simulink model "BMS_System_Arch"  (R2024a)
settings: Solver=VariableStepAuto  StartTime=0.0  StopTime=10.0  RelTol=1e-3
settings Model: DataDictionary=BMS_System_Arch_dict.sldd  Creator=ghourabi  LastModifiedBy=hirah

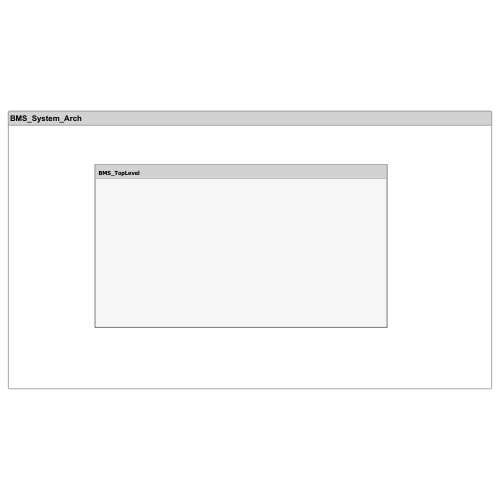
[thumbnail: Simulink's stored preview of the top-level diagram]
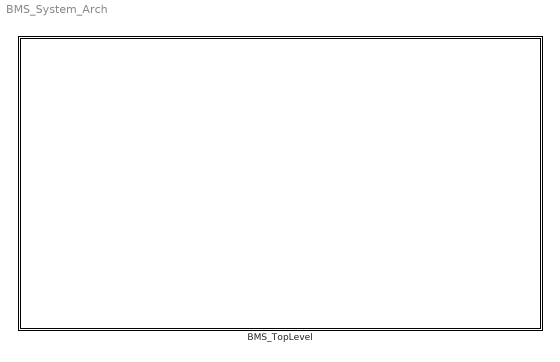
== system BMS_System_Arch ==
  "BMS_TopLevel " : Subsystem
      settings: PortSchema="{\"entries\":[{\"content\":{\"headerSize\":26,\"margin\":15,\"minimumSpacing\":25,\"sides\":[{\"content\":{},\"type\":\"ConnectorPlacement.EquallySpacedRectSide\",\"uuid\":\"3cb385af-e70b-4c78-b84b-8b5b4c1bf807\"},{\"content\":{\"side\":\"RIGHT\"},\"type\":\"ConnectorPlacement.EquallySpacedRectSide\",\"uuid\":\"e6b0f49b-5901-429a-bf04-96c47fe1d754\"},{\"content\":{\"side\":\"TOP\"},\"type\":\"ConnectorPlacement.EquallySpacedRectSide\",\"uuid\":\"0aec474f-0a8e-4cc4-a707-3f6b1e91156f\"}]},\"type\":\"ConnectorPlacement.EquallySpacedConnector\",\"uuid\":\"d23b7e1f-ccd0-4a91-b27d-bb01c8043b47\"}],\"packageUris\":[\"http://schema.mathworks.com/mf0/Connector/R2020b\"],\"version\":\"1.0\"}"

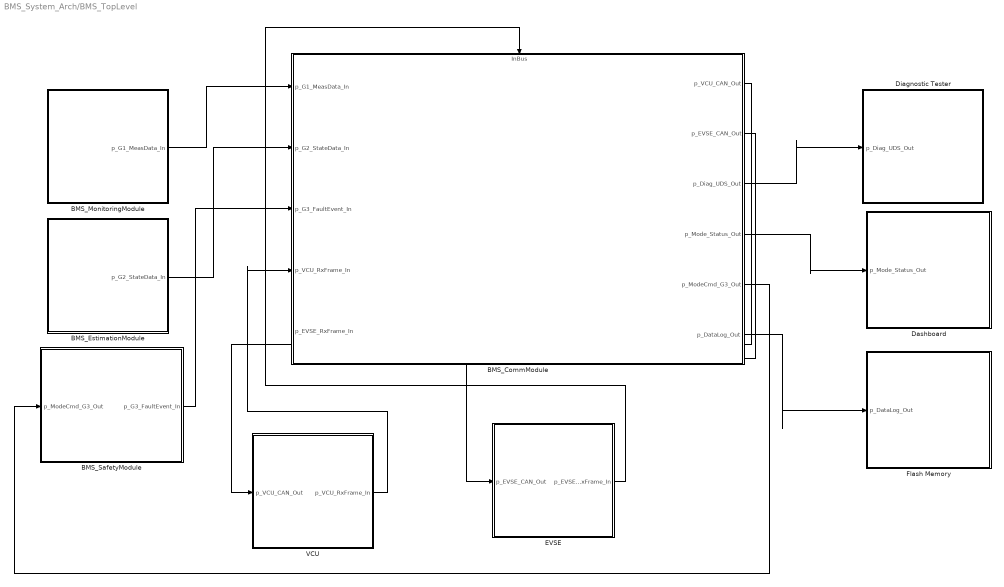
== system BMS_System_Arch/BMS_TopLevel  ==
  BMS_CommModule : Subsystem
      settings: PortSchema="{\"entries\":[{\"content\":{\"headerSize\":26,\"margin\":15,\"minimumSpacing\":25,\"sides\":[{\"content\":{\"connectorIds\":[\"In2\",\"In3\",\"In4\",\"In5\",\"In6\"]},\"type\":\"ConnectorPlacement.EquallySpacedRectSide\",\"uuid\":\"3cb385af-e70b-4c78-b84b-8b5b4c1bf807\"},{\"content\":{\"connectorIds\":[\"Out1\",\"Out2\",\"Out3\",\"Out4\",\"Out5\",\"Out6\"],\"side\":\"RIGHT\"},\"type\":\"ConnectorPlacement.EquallySpacedRectSide\",\"uuid\":\"e6b0f49b-5901-429a-bf04-96c47fe1d754\"},{\"content\":{\"connectorIds\":[\"In1\"],\"side\":\"TOP\"},\"type\":\"ConnectorPlacement.EquallySpacedRectSide\",\"uuid\":\"0aec474f-0a8e-4cc4-a707-3f6b1e91156f\"}]},\"type\":\"ConnectorPlacement.EquallySpacedConnector\",\"uuid\":\"d23b7e1f-ccd0-4a91-b27d-bb01c8043b47\"}],\"packageUris\":[\"http://schema.mathworks.com/mf0/Connector/R2020b\"],\"version\":\"1.0\"}"
  BMS_EstimationModule : Subsystem
      settings: PortSchema="{\"entries\":[{\"content\":{\"headerSize\":26,\"margin\":15,\"minimumSpacing\":25,\"sides\":[{\"content\":{},\"type\":\"ConnectorPlacement.EquallySpacedRectSide\",\"uuid\":\"3cb385af-e70b-4c78-b84b-8b5b4c1bf807\"},{\"content\":{\"connectorIds\":[\"Out1\"],\"side\":\"RIGHT\"},\"type\":\"ConnectorPlacement.EquallySpacedRectSide\",\"uuid\":\"e6b0f49b-5901-429a-bf04-96c47fe1d754\"},{\"content\":{\"side\":\"TOP\"},\"type\":\"ConnectorPlacement.EquallySpacedRectSide\",\"uuid\":\"0aec474f-0a8e-4cc4-a707-3f6b1e91156f\"}]},\"type\":\"ConnectorPlacement.EquallySpacedConnector\",\"uuid\":\"d23b7e1f-ccd0-4a91-b27d-bb01c8043b47\"}],\"packageUris\":[\"http://schema.mathworks.com/mf0/Connector/R2020b\"],\"version\":\"1.0\"}"
  BMS_MonitoringModule : Subsystem
      settings: PortSchema="{\"entries\":[{\"content\":{\"headerSize\":26,\"margin\":15,\"minimumSpacing\":25,\"sides\":[{\"content\":{},\"type\":\"ConnectorPlacement.EquallySpacedRectSide\",\"uuid\":\"3cb385af-e70b-4c78-b84b-8b5b4c1bf807\"},{\"content\":{\"connectorIds\":[\"Out1\"],\"side\":\"RIGHT\"},\"type\":\"ConnectorPlacement.EquallySpacedRectSide\",\"uuid\":\"e6b0f49b-5901-429a-bf04-96c47fe1d754\"},{\"content\":{\"side\":\"TOP\"},\"type\":\"ConnectorPlacement.EquallySpacedRectSide\",\"uuid\":\"0aec474f-0a8e-4cc4-a707-3f6b1e91156f\"}]},\"type\":\"ConnectorPlacement.EquallySpacedConnector\",\"uuid\":\"d23b7e1f-ccd0-4a91-b27d-bb01c8043b47\"}],\"packageUris\":[\"http://schema.mathworks.com/mf0/Connector/R2020b\"],\"version\":\"1.0\"}"
  BMS_SafetyModule : Subsystem
      settings: PortSchema="{\"entries\":[{\"content\":{\"headerSize\":26,\"margin\":15,\"minimumSpacing\":25,\"sides\":[{\"content\":{\"connectorIds\":[\"In1\"]},\"type\":\"ConnectorPlacement.EquallySpacedRectSide\",\"uuid\":\"3cb385af-e70b-4c78-b84b-8b5b4c1bf807\"},{\"content\":{\"connectorIds\":[\"Out1\"],\"side\":\"RIGHT\"},\"type\":\"ConnectorPlacement.EquallySpacedRectSide\",\"uuid\":\"e6b0f49b-5901-429a-bf04-96c47fe1d754\"},{\"content\":{\"side\":\"TOP\"},\"type\":\"ConnectorPlacement.EquallySpacedRectSide\",\"uuid\":\"0aec474f-0a8e-4cc4-a707-3f6b1e91156f\"}]},\"type\":\"ConnectorPlacement.EquallySpacedConnector\",\"uuid\":\"d23b7e1f-ccd0-4a91-b27d-bb01c8043b47\"}],\"packageUris\":[\"http://schema.mathworks.com/mf0/Connector/R2020b\"],\"version\":\"1.0\"}"
  "Dashboard " : Subsystem
      settings: PortSchema="{\"entries\":[{\"content\":{\"headerSize\":26,\"margin\":15,\"minimumSpacing\":25,\"sides\":[{\"content\":{\"connectorIds\":[\"In1\"]},\"type\":\"ConnectorPlacement.EquallySpacedRectSide\",\"uuid\":\"3cb385af-e70b-4c78-b84b-8b5b4c1bf807\"},{\"content\":{\"side\":\"RIGHT\"},\"type\":\"ConnectorPlacement.EquallySpacedRectSide\",\"uuid\":\"e6b0f49b-5901-429a-bf04-96c47fe1d754\"},{\"content\":{\"side\":\"TOP\"},\"type\":\"ConnectorPlacement.EquallySpacedRectSide\",\"uuid\":\"0aec474f-0a8e-4cc4-a707-3f6b1e91156f\"}]},\"type\":\"ConnectorPlacement.EquallySpacedConnector\",\"uuid\":\"d23b7e1f-ccd0-4a91-b27d-bb01c8043b47\"}],\"packageUris\":[\"http://schema.mathworks.com/mf0/Connector/R2020b\"],\"version\":\"1.0\"}"
  "Diagnostic Tester " : Subsystem
      settings: PortSchema="{\"entries\":[{\"content\":{\"headerSize\":26,\"margin\":15,\"minimumSpacing\":25,\"sides\":[{\"content\":{\"connectorIds\":[\"In1\"]},\"type\":\"ConnectorPlacement.EquallySpacedRectSide\",\"uuid\":\"3cb385af-e70b-4c78-b84b-8b5b4c1bf807\"},{\"content\":{\"side\":\"RIGHT\"},\"type\":\"ConnectorPlacement.EquallySpacedRectSide\",\"uuid\":\"e6b0f49b-5901-429a-bf04-96c47fe1d754\"},{\"content\":{\"side\":\"TOP\"},\"type\":\"ConnectorPlacement.EquallySpacedRectSide\",\"uuid\":\"0aec474f-0a8e-4cc4-a707-3f6b1e91156f\"}]},\"type\":\"ConnectorPlacement.EquallySpacedConnector\",\"uuid\":\"d23b7e1f-ccd0-4a91-b27d-bb01c8043b47\"}],\"packageUris\":[\"http://schema.mathworks.com/mf0/Connector/R2020b\"],\"version\":\"1.0\"}"
  "EVSE " : Subsystem
      settings: PortSchema="{\"entries\":[{\"content\":{\"headerSize\":26,\"margin\":15,\"minimumSpacing\":25,\"sides\":[{\"content\":{\"connectorIds\":[\"In1\"]},\"type\":\"ConnectorPlacement.EquallySpacedRectSide\",\"uuid\":\"3cb385af-e70b-4c78-b84b-8b5b4c1bf807\"},{\"content\":{\"connectorIds\":[\"Out1\"],\"side\":\"RIGHT\"},\"type\":\"ConnectorPlacement.EquallySpacedRectSide\",\"uuid\":\"e6b0f49b-5901-429a-bf04-96c47fe1d754\"},{\"content\":{\"side\":\"TOP\"},\"type\":\"ConnectorPlacement.EquallySpacedRectSide\",\"uuid\":\"0aec474f-0a8e-4cc4-a707-3f6b1e91156f\"}]},\"type\":\"ConnectorPlacement.EquallySpacedConnector\",\"uuid\":\"d23b7e1f-ccd0-4a91-b27d-bb01c8043b47\"}],\"packageUris\":[\"http://schema.mathworks.com/mf0/Connector/R2020b\"],\"version\":\"1.0\"}"
  "Flash Memory " : Subsystem
      settings: PortSchema="{\"entries\":[{\"content\":{\"headerSize\":26,\"margin\":15,\"minimumSpacing\":25,\"sides\":[{\"content\":{\"connectorIds\":[\"In1\"]},\"type\":\"ConnectorPlacement.EquallySpacedRectSide\",\"uuid\":\"3cb385af-e70b-4c78-b84b-8b5b4c1bf807\"},{\"content\":{\"side\":\"RIGHT\"},\"type\":\"ConnectorPlacement.EquallySpacedRectSide\",\"uuid\":\"e6b0f49b-5901-429a-bf04-96c47fe1d754\"},{\"content\":{\"side\":\"TOP\"},\"type\":\"ConnectorPlacement.EquallySpacedRectSide\",\"uuid\":\"0aec474f-0a8e-4cc4-a707-3f6b1e91156f\"}]},\"type\":\"ConnectorPlacement.EquallySpacedConnector\",\"uuid\":\"d23b7e1f-ccd0-4a91-b27d-bb01c8043b47\"}],\"packageUris\":[\"http://schema.mathworks.com/mf0/Connector/R2020b\"],\"version\":\"1.0\"}"
  VCU : Subsystem
      settings: PortSchema="{\"entries\":[{\"content\":{\"headerSize\":26,\"margin\":15,\"minimumSpacing\":25,\"sides\":[{\"content\":{\"connectorIds\":[\"In1\"]},\"type\":\"ConnectorPlacement.EquallySpacedRectSide\",\"uuid\":\"3cb385af-e70b-4c78-b84b-8b5b4c1bf807\"},{\"content\":{\"connectorIds\":[\"Out1\"],\"side\":\"RIGHT\"},\"type\":\"ConnectorPlacement.EquallySpacedRectSide\",\"uuid\":\"e6b0f49b-5901-429a-bf04-96c47fe1d754\"},{\"content\":{\"side\":\"TOP\"},\"type\":\"ConnectorPlacement.EquallySpacedRectSide\",\"uuid\":\"0aec474f-0a8e-4cc4-a707-3f6b1e91156f\"}]},\"type\":\"ConnectorPlacement.EquallySpacedConnector\",\"uuid\":\"d23b7e1f-ccd0-4a91-b27d-bb01c8043b47\"}],\"packageUris\":[\"http://schema.mathworks.com/mf0/Connector/R2020b\"],\"version\":\"1.0\"}"
  wires:
  BMS_MonitoringModule/1(p_G1_MeasData_In) -> BMS_CommModule/2(p_G1_MeasData_In)
  BMS_EstimationModule/1(p_G2_StateData_In) -> BMS_CommModule/3(p_G2_StateData_In)
  BMS_SafetyModule/1(p_G3_FaultEvent_In) -> BMS_CommModule/4(p_G3_FaultEvent_In)
  VCU/1(p_VCU_RxFrame_In) -> BMS_CommModule/5(p_VCU_RxFrame_In)
  "EVSE "/1(p_EVSE_RxFrame_In) -> BMS_CommModule/1(InBus)
  BMS_CommModule/1(p_VCU_CAN_Out) -> VCU/1(p_VCU_CAN_Out)
  BMS_CommModule/2(p_EVSE_CAN_Out) -> "EVSE "/1(p_EVSE_CAN_Out)
  BMS_CommModule/3(p_Diag_UDS_Out) -> "Diagnostic Tester "/1(p_Diag_UDS_Out)
  BMS_CommModule/4(p_Mode_Status_Out) -> "Dashboard "/1(p_Mode_Status_Out)
  BMS_CommModule/6(p_DataLog_Out) -> "Flash Memory "/1(p_DataLog_Out)
  BMS_CommModule/5(p_ModeCmd_G3_Out) -> BMS_SafetyModule/1(p_ModeCmd_G3_Out)

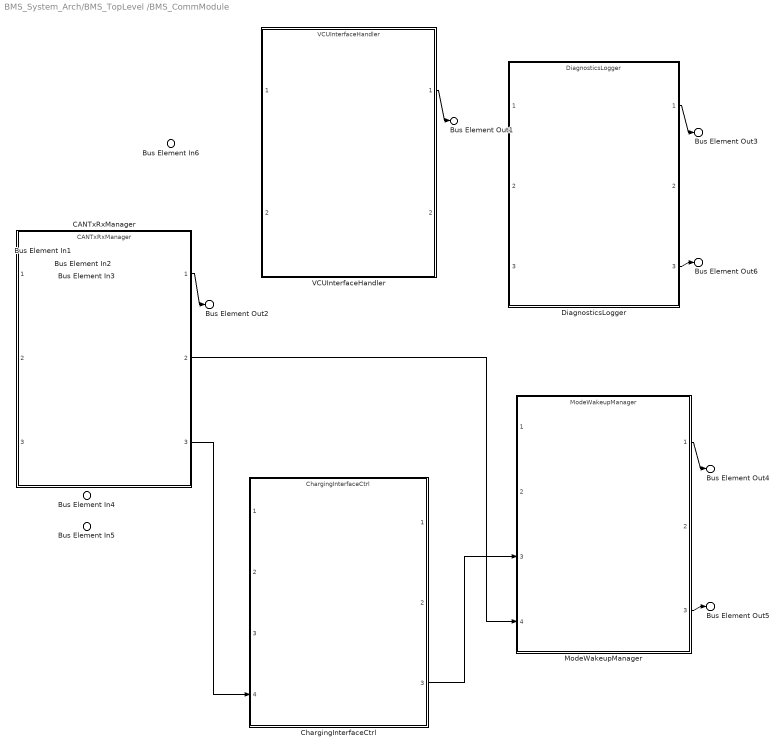
== system BMS_System_Arch/BMS_TopLevel /BMS_CommModule ==
  Bus Element In6 : Inport  PortName=InBus
  Bus Element In1 : Inport  Port=2  PortName=p_G1_MeasData_In
  Bus Element In2 : Inport  Port=3  PortName=p_G2_StateData_In
  Bus Element In3 : Inport  Port=4  PortName=p_G3_FaultEvent_In
  Bus Element In4 : Inport  Port=5  PortName=p_VCU_RxFrame_In
  Bus Element In5 : Inport  Port=6  PortName=p_EVSE_RxFrame_In
  CANTxRxManager : ModelReference  ModelNameDialog=CANTxRxManager  SimulationMode=Normal  ModelReferenceVersion=1.3
      settings: PortSchema="{\"entries\":[{\"content\":{\"headerSize\":38,\"margin\":15,\"minimumSpacing\":25,\"sides\":[{\"content\":{\"connectorIds\":[\"In1\",\"In2\",\"In3\"]},\"type\":\"ConnectorPlacement.EquallySpacedRectSide\",\"uuid\":\"3cb385af-e70b-4c78-b84b-8b5b4c1bf807\"},{\"content\":{\"connectorIds\":[\"Out1\",\"Out2\",\"Out3\"],\"side\":\"RIGHT\"},\"type\":\"ConnectorPlacement.EquallySpacedRectSide\",\"uuid\":\"e6b0f49b-5901-429a-bf04-96c47fe1d754\"},{\"content\":{\"side\":\"TOP\"},\"type\":\"ConnectorPlacement.EquallySpacedRectSide\",\"uuid\":\"0aec474f-0a8e-4cc4-a707-3f6b1e91156f\"}]},\"type\":\"ConnectorPlacement.EquallySpacedConnector\",\"uuid\":\"d23b7e1f-ccd0-4a91-b27d-bb01c8043b47\"}],\"packageUris\":[\"http://schema.mathworks.com/mf0/Connector/R2020b\"],\"version\":\"1.0\"}"
  "ChargingInterfaceCtrl " : ModelReference  ModelNameDialog=ChargingInterfaceCtrl  SimulationMode=Normal  ModelReferenceVersion=1.7
      settings: PortSchema="{\"entries\":[{\"content\":{\"headerSize\":38,\"margin\":15,\"minimumSpacing\":25,\"sides\":[{\"content\":{\"connectorIds\":[\"In1\",\"In2\",\"In3\",\"In4\"]},\"type\":\"ConnectorPlacement.EquallySpacedRectSide\",\"uuid\":\"3cb385af-e70b-4c78-b84b-8b5b4c1bf807\"},{\"content\":{\"connectorIds\":[\"Out1\",\"Out2\",\"Out3\"],\"side\":\"RIGHT\"},\"type\":\"ConnectorPlacement.EquallySpacedRectSide\",\"uuid\":\"e6b0f49b-5901-429a-bf04-96c47fe1d754\"},{\"content\":{\"side\":\"TOP\"},\"type\":\"ConnectorPlacement.EquallySpacedRectSide\",\"uuid\":\"0aec474f-0a8e-4cc4-a707-3f6b1e91156f\"}]},\"type\":\"ConnectorPlacement.EquallySpacedConnector\",\"uuid\":\"d23b7e1f-ccd0-4a91-b27d-bb01c8043b47\"}],\"packageUris\":[\"http://schema.mathworks.com/mf0/Connector/R2020b\"],\"version\":\"1.0\"}"
  "DiagnosticsLogger " : ModelReference  ModelNameDialog=DiagnosticsLogger  SimulationMode=Normal  ModelReferenceVersion=1.2
      settings: PortSchema="{\"entries\":[{\"content\":{\"headerSize\":38,\"margin\":15,\"minimumSpacing\":25,\"sides\":[{\"content\":{\"connectorIds\":[\"In1\",\"In2\",\"In3\"]},\"type\":\"ConnectorPlacement.EquallySpacedRectSide\",\"uuid\":\"3cb385af-e70b-4c78-b84b-8b5b4c1bf807\"},{\"content\":{\"connectorIds\":[\"Out1\",\"Out2\",\"Out3\"],\"side\":\"RIGHT\"},\"type\":\"ConnectorPlacement.EquallySpacedRectSide\",\"uuid\":\"e6b0f49b-5901-429a-bf04-96c47fe1d754\"},{\"content\":{\"side\":\"TOP\"},\"type\":\"ConnectorPlacement.EquallySpacedRectSide\",\"uuid\":\"0aec474f-0a8e-4cc4-a707-3f6b1e91156f\"}]},\"type\":\"ConnectorPlacement.EquallySpacedConnector\",\"uuid\":\"d23b7e1f-ccd0-4a91-b27d-bb01c8043b47\"}],\"packageUris\":[\"http://schema.mathworks.com/mf0/Connector/R2020b\"],\"version\":\"1.0\"}"
  "ModeWakeupManager " : ModelReference  ModelNameDialog=ModeWakeupManager  SimulationMode=Normal  ModelReferenceVersion=1.4
      settings: PortSchema="{\"entries\":[{\"content\":{\"headerSize\":38,\"margin\":15,\"minimumSpacing\":25,\"sides\":[{\"content\":{\"connectorIds\":[\"In1\",\"In2\",\"In3\",\"In4\"]},\"type\":\"ConnectorPlacement.EquallySpacedRectSide\",\"uuid\":\"3cb385af-e70b-4c78-b84b-8b5b4c1bf807\"},{\"content\":{\"connectorIds\":[\"Out1\",\"Out2\",\"Out3\"],\"side\":\"RIGHT\"},\"type\":\"ConnectorPlacement.EquallySpacedRectSide\",\"uuid\":\"e6b0f49b-5901-429a-bf04-96c47fe1d754\"},{\"content\":{\"side\":\"TOP\"},\"type\":\"ConnectorPlacement.EquallySpacedRectSide\",\"uuid\":\"0aec474f-0a8e-4cc4-a707-3f6b1e91156f\"}]},\"type\":\"ConnectorPlacement.EquallySpacedConnector\",\"uuid\":\"d23b7e1f-ccd0-4a91-b27d-bb01c8043b47\"}],\"packageUris\":[\"http://schema.mathworks.com/mf0/Connector/R2020b\"],\"version\":\"1.0\"}"
  VCUInterfaceHandler : ModelReference  ModelNameDialog=VCUInterfaceHandler  SimulationMode=Normal  ModelReferenceVersion=1.3
      settings: PortSchema="{\"entries\":[{\"content\":{\"headerSize\":38,\"margin\":15,\"minimumSpacing\":25,\"sides\":[{\"content\":{\"connectorIds\":[\"In1\",\"In2\"]},\"type\":\"ConnectorPlacement.EquallySpacedRectSide\",\"uuid\":\"3cb385af-e70b-4c78-b84b-8b5b4c1bf807\"},{\"content\":{\"connectorIds\":[\"Out1\",\"Out2\"],\"side\":\"RIGHT\"},\"type\":\"ConnectorPlacement.EquallySpacedRectSide\",\"uuid\":\"e6b0f49b-5901-429a-bf04-96c47fe1d754\"},{\"content\":{\"side\":\"TOP\"},\"type\":\"ConnectorPlacement.EquallySpacedRectSide\",\"uuid\":\"0aec474f-0a8e-4cc4-a707-3f6b1e91156f\"}]},\"type\":\"ConnectorPlacement.EquallySpacedConnector\",\"uuid\":\"d23b7e1f-ccd0-4a91-b27d-bb01c8043b47\"}],\"packageUris\":[\"http://schema.mathworks.com/mf0/Connector/R2020b\"],\"version\":\"1.0\"}"
  Bus Element Out1 : Outport  PortName=p_VCU_CAN_Out
  Bus Element Out2 : Outport  Port=2  PortName=p_EVSE_CAN_Out
  Bus Element Out3 : Outport  Port=3  PortName=p_Diag_UDS_Out
  Bus Element Out4 : Outport  Port=4  PortName=p_Mode_Status_Out
  Bus Element Out5 : Outport  Port=5  PortName=p_ModeCmd_G3_Out
  Bus Element Out6 : Outport  Port=6  PortName=p_DataLog_Out
  wires:
  CANTxRxManager/1 -> Bus Element Out2/1
  VCUInterfaceHandler/1 -> Bus Element Out1/1
  "DiagnosticsLogger "/3 -> Bus Element Out6/1
  "DiagnosticsLogger "/1 -> Bus Element Out3/1
  CANTxRxManager/3 -> "ChargingInterfaceCtrl "/4
  "ChargingInterfaceCtrl "/3 -> "ModeWakeupManager "/3
  CANTxRxManager/2 -> "ModeWakeupManager "/4
  "ModeWakeupManager "/1 -> Bus Element Out4/1
  "ModeWakeupManager "/3 -> Bus Element Out5/1

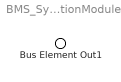
== system BMS_System_Arch/BMS_TopLevel /BMS_EstimationModule ==
  Bus Element Out1 : Outport  PortName=p_G2_StateData_In

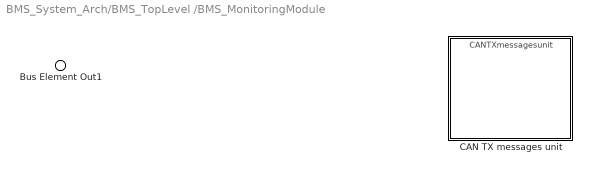
== system BMS_System_Arch/BMS_TopLevel /BMS_MonitoringModule ==
  CAN TX messages unit : ModelReference  ModelNameDialog=CANTXmessagesunit  SimulationMode=Normal  ModelReferenceVersion=1.1
      settings: PortSchema="{\"entries\":[{\"content\":{\"headerSize\":38,\"margin\":15,\"minimumSpacing\":25,\"sides\":[{\"content\":{},\"type\":\"ConnectorPlacement.EquallySpacedRectSide\",\"uuid\":\"5bf11642-2165-495a-8f16-07288b1b2a7f\"},{\"content\":{\"side\":\"RIGHT\"},\"type\":\"ConnectorPlacement.EquallySpacedRectSide\",\"uuid\":\"16013c05-30c7-4811-aab5-6705354ddbd6\"},{\"content\":{\"side\":\"TOP\"},\"type\":\"ConnectorPlacement.EquallySpacedRectSide\",\"uuid\":\"95109c83-3f97-4257-a072-0eae8b681641\"}]},\"type\":\"ConnectorPlacement.EquallySpacedConnector\",\"uuid\":\"ab507b5d-7f02-463f-8b22-b752f4ca7c99\"}],\"packageUris\":[\"http://schema.mathworks.com/mf0/Connector/R2020b\"],\"version\":\"1.0\"}"
  Bus Element Out1 : Outport  PortName=p_G1_MeasData_In

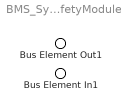
== system BMS_System_Arch/BMS_TopLevel /BMS_SafetyModule ==
  Bus Element In1 : Inport  PortName=p_ModeCmd_G3_Out
  Bus Element Out1 : Outport  PortName=p_G3_FaultEvent_In

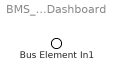
== system BMS_System_Arch/BMS_TopLevel /Dashboard  ==
  Bus Element In1 : Inport  PortName=p_Mode_Status_Out

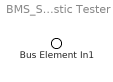
== system BMS_System_Arch/BMS_TopLevel /Diagnostic Tester  ==
  Bus Element In1 : Inport  PortName=p_Diag_UDS_Out

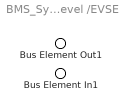
== system BMS_System_Arch/BMS_TopLevel /EVSE  ==
  Bus Element In1 : Inport  PortName=p_EVSE_CAN_Out
  Bus Element Out1 : Outport  PortName=p_EVSE_RxFrame_In

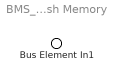
== system BMS_System_Arch/BMS_TopLevel /Flash Memory  ==
  Bus Element In1 : Inport  PortName=p_DataLog_Out

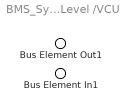
== system BMS_System_Arch/BMS_TopLevel /VCU ==
  Bus Element In1 : Inport  PortName=p_VCU_CAN_Out
  Bus Element Out1 : Outport  PortName=p_VCU_RxFrame_In
